simulink model "CA2_2"  (R2023b)
settings: Solver=VariableStepAuto  StartTime=0.0  StopTime=10.0  RelTol=1e-3
settings Model: Creator=shipingguo  LastModifiedBy=shipingguo
settings SolverCC: ZeroCrossAlgorithm=Adaptive
settings DebuggingCC: IgnoredZcDiagnostic=none

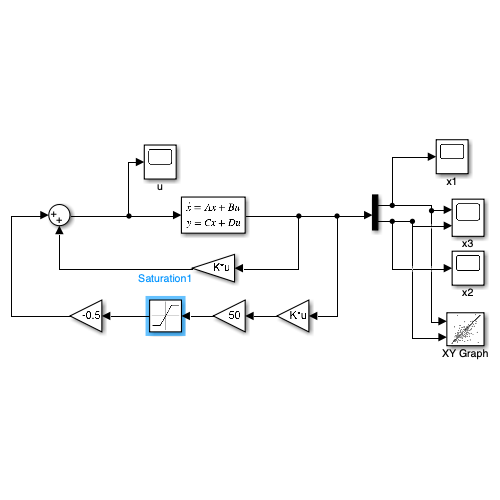
[thumbnail: Simulink's stored preview of the top-level diagram]
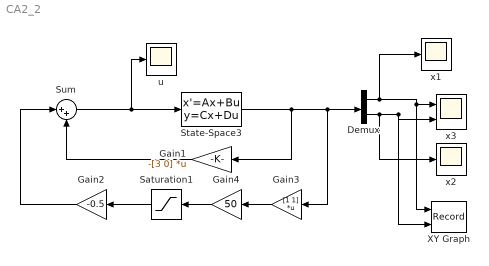
== system CA2_2 ==
  Demux : Demux  Outputs=2
  Gain1 : Gain  Gain=-[3 0]  Multiplication=Matrix(K*u)
  Gain2 : Gain  Gain=-0.5
  Gain3 : Gain  Gain=[1 1]  Multiplication=Matrix(K*u)
  Gain4 : Gain  Gain=50
  Saturation1 : Saturate  UpperLimit=1  LowerLimit=-1
  State-Space3 : StateSpace  A=[1 0; 1 0]  B=[1; 0]  C=[1 0; 0 1]  D=[0 ; 0 ]  InitialCondition=[1.5; 0]
  Sum : Sum  Inputs=|++
  XY Graph : Record  FileSettingsInternal="{\"entries\":[{\"content\":{\"excelSettings\":{\"content\":{},\"type\":\"Streamout.ExcelSettings\"}},\"type\":\"Streamout.FileSettingStorage\",\"uuid\":\"\"}],\"packageUris\":[\"http:\\/\\/schema.mathworks.com\\/mf0\\/streamout_blocks\\/R2020a\"],\"version\":\"1.0\"}"  Layout=[1 1]  SignalsInternal="{\"entries\":[{\"content\":{\"signals\":[{\"content\":{\"blockPath\":[],\"dimensions\":[1],\"domain\":\"\",\"lineColor\":\"#a2142f\",\"plots\":[1],\"port\":1,\"sid\":[\"\"],\"signalID\":491,\"signalName\":\"Demux:1\"},\"type\":\"RecordBlkView.Signal\",\"uuid\":\"\"},{\"content\":{\"blockPath\":[],\"dimensions\":[1],\"domain\":\"\",\"lineColor\":\"#139fff\",\"plots\":[1],\"port\":2,\"sid\":[\"\"],\"signalID\":495,\"signalName\":\"Demux:2\"},\"type\":\"RecordBlkView.Signal\",\"uuid\":\"\"}]},\"type\":\"RecordBlkView.InputSignals\",\"uuid\":\"\"}],\"packageUris\":[\"http:\\/\\/schema.mathworks.com\\/mf0\\/streamout_blocks\\/R2020a\"],\"version\":\"1.0\"}"  VisualizationBindings="{\"xyplotplugin\":{\"info\":[{\"series\":[{\"bindingParametersList\":[{\"parameter\":\"X-Axis\",\"signalID\":491,\"signalName\":\"Demux:1\"},{\"parameter\":\"Y-Axis\",\"signalID\":495,\"signalName\":\"Demux:2\"}],\"seriesID\":27117}],\"subplotID\":1}]}}"  CompatibilityTag=XY
  u : Scope
  x1 : Scope
  x2 : Scope
  x3 : Scope  NumInputPorts=2
  wires:
  Gain1/1 -> Sum/2
  Saturation1/1 -> Gain2/1
  Gain2/1 -> Sum/1
  Sum/1 -> u/1, State-Space3/1
  State-Space3/1 -> Gain1/1, Gain3/1, Demux/1
  Demux/1 -> x1/1, XY Graph/1, x3/1
  Demux/2 -> x3/2, XY Graph/2, x2/1
  Gain4/1 -> Saturation1/1
  Gain3/1 -> Gain4/1
